simulink library "INT_CoVMD_TrqCalc"  (R2016b)
settings: Solver=VariableStepAuto  StartTime=0.0  StopTime=10.0  RelTol=1e-3
settings Model: Creator=Administrator  LastModifiedBy=Administrator

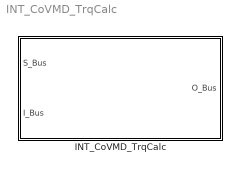
== system INT_CoVMD_TrqCalc ==
  INT_CoVMD_TrqCalc : Subsystem

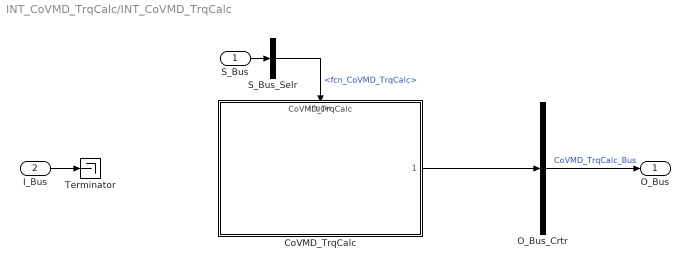
== system INT_CoVMD_TrqCalc/INT_CoVMD_TrqCalc ==
  S_Bus : Inport
  I_Bus : Inport  Port=2
  CoVMD_TrqCalc : ModelReference  ModelNameDialog=CoVMD_TrqCalc  SimulationMode=Normal  ModelReferenceVersion=1.2  TriggerPortName=function  TriggerPortTriggerType=function-call  TriggerPortStatesWhenEnabling=held
  O_Bus_Crtr : BusCreator  Inputs=1
  S_Bus_Selr : BusSelector  OutputSignals=fcn_CoVMD_TrqCalc
  Terminator : Terminator
  O_Bus : Outport
  wires:
  S_Bus_Selr/1 -> CoVMD_TrqCalc/Trigger  "<fcn_CoVMD_TrqCalc>"
  S_Bus/1 -> S_Bus_Selr/1
  I_Bus/1 -> Terminator/1
  O_Bus_Crtr/1 -> O_Bus/1  "CoVMD_TrqCalc_Bus"
  CoVMD_TrqCalc/1 -> O_Bus_Crtr/1
